simulink model "funkcia2"  (R2020a)
settings: Solver=VariableStepAuto  StartTime=0.0  StopTime=10.0  RelTol=1e-3
libraries: simulink x1
settings Model: Creator=xacha  LastModifiedBy=xacha

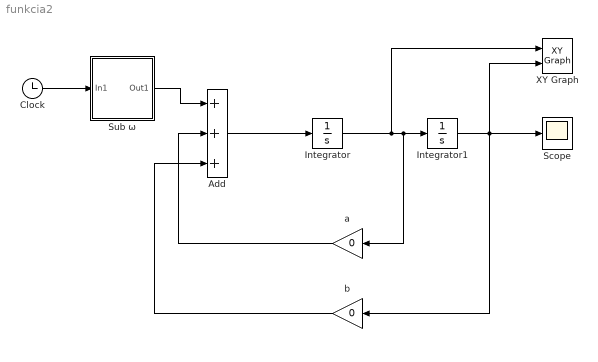
== system funkcia2 ==
  Add : Sum  Inputs=+++
  Clock : Clock
  Integrator : Integrator
  Integrator1 : Integrator
  Scope : Scope
  "Sub ω " : Subsystem  mask{a=1}
      mask prompts: a "input a"
  XY Graph : simulink/Sinks/XY Graph  xmin=-1  xmax=1  ymin=-1  ymax=1  st=-1
  a : Gain  Gain=0  mask{a=0}
      mask prompts: a "input a"
  b : Gain  Gain=0  mask{b=1}
      mask prompts: b "input b"
  wires:
  Integrator/1 -> XY Graph/1, a/1, Integrator1/1
  a/1 -> Add/2
  Clock/1 -> "Sub ω "/1(In1)
  Integrator1/1 -> b/1, XY Graph/2, Scope/1
  Add/1 -> Integrator/1
  "Sub ω "/1(Out1) -> Add/1
  b/1 -> Add/3

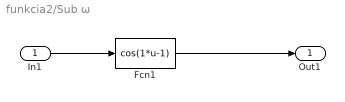
== system funkcia2/Sub ω  ==
  In1 : Inport
  Fcn1 : Fcn  Expr=cos(1*u-1)
  Out1 : Outport  VectorParamsAs1DForOutWhenUnconnected=off
  wires:
  In1/1 -> Fcn1/1
  Fcn1/1 -> Out1/1
